simulink model "PESO_ex1"  (R2020b)
settings: Solver=VariableStepAuto  StartTime=0.0  StopTime=20  FixedStep=1e-6  RelTol=1e-4
settings Model: Creator=Amir  LastModifiedBy=Amir
settings DataIOCC: ReturnWorkspaceOutputs=off

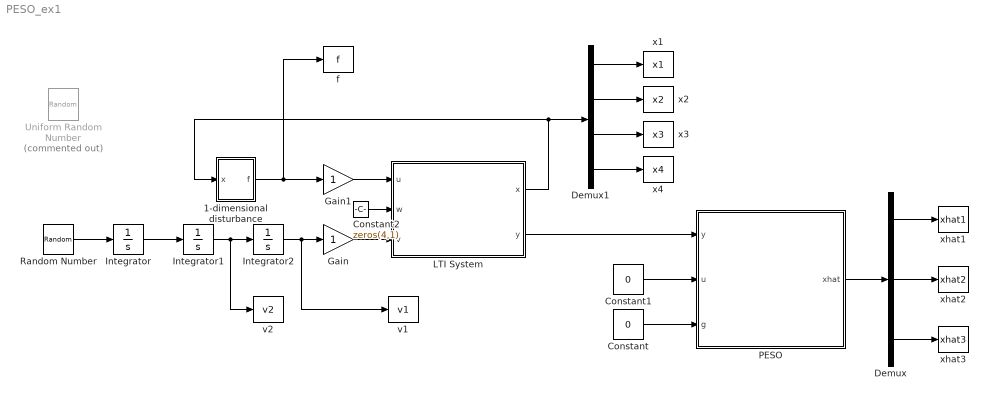
== system PESO_ex1 ==
  1-dimensional disturbance : Subsystem
  Constant : Constant  Value=0
  Constant1 : Constant  Value=0
  Constant2 : Constant  Value=zeros(4,1)
  Demux : Demux  Outputs=3
  Demux1 : Demux
  Gain : Gain
  Gain1 : Gain
  Integrator : Integrator
  Integrator1 : Integrator
  Integrator2 : Integrator
  LTI System : Subsystem  mask{n=4, m=1, k=1, A=[0 1 0 0;0 0 1 0;0 0 0 1;0 0 0 0], B=[0;0;0;1], C=[1 0 0 0], D=0, x0=[1;1;1;1]}
      mask prompts: n "Length of state vector (n):"; m "Length of input vector (m):"; k "Length of output vector (k):"; x0 "x(0):"
      mask DialogControl DescGroupVar Prompt: Main
      mask DialogControl DescTextVar Prompt: This block simulates a linear time-invariant (LTI) system. The system can be written as 'dx/dt=Ax+Bu+w' and 'y=Cx+Du+v'.
      mask DialogControl ParameterGroupVar Prompt: Dimensions
      mask DialogControl ParameterGroupVar_copy Prompt: Parameters
      mask DialogControl ParameterGroupVar_copy_copy Prompt: Initial Condition
  PESO : Subsystem  mask{n=2, tau=20, b=-[3;3;1], alpha=0.03, x0=10*[1;1], epsilon_t=1e-3}
      mask prompts: n "Dimension of the system (n):"; tau "Convergence time (tau):"; b "Vector of observer gains (b):"; alpha "Mapping gain (alpha):"; x0 "Initial Estimated state (x0):"; epsilon_t "Switching tolerance (epsilon_t):"
      mask DialogControl DescGroupVar Prompt: Main
      mask DialogControl DescTextVar Prompt: Prescribed-time observer for unknown systems.
  Random Number : RandomNumber  Variance=1e-6  SampleTime=1e-4
  Uniform Random Number : UniformRandomNumber  Commented=on  Minimum=-1e-3  Maximum=1e-3  Seed=-100  SampleTime=1e-4
  f : ToWorkspace  VariableName=f  SampleTime=-1
      settings: Save2DSignal=2-D array (concatenate along first dimension)
  v1 : ToWorkspace  VariableName=v1  SampleTime=-1
      settings: Save2DSignal=2-D array (concatenate along first dimension)
  v2 : ToWorkspace  VariableName=v2  SampleTime=-1
      settings: Save2DSignal=2-D array (concatenate along first dimension)
  x1 : ToWorkspace  VariableName=x1  SampleTime=-1
      settings: Save2DSignal=2-D array (concatenate along first dimension)
  x2 : ToWorkspace  VariableName=x2  SampleTime=-1
      settings: Save2DSignal=2-D array (concatenate along first dimension)
  x3 : ToWorkspace  VariableName=x3  SampleTime=-1
      settings: Save2DSignal=2-D array (concatenate along first dimension)
  x4 : ToWorkspace  VariableName=x4  SampleTime=-1
      settings: Save2DSignal=2-D array (concatenate along first dimension)
  xhat1 : ToWorkspace  VariableName=xhat1  SampleTime=-1
      settings: Save2DSignal=2-D array (concatenate along first dimension)
  xhat2 : ToWorkspace  VariableName=xhat2  SampleTime=-1
      settings: Save2DSignal=2-D array (concatenate along first dimension)
  xhat3 : ToWorkspace  VariableName=xhat3  SampleTime=-1
      settings: Save2DSignal=2-D array (concatenate along first dimension)
  wires:
  LTI System/2(y) -> PESO/1(y)
  PESO/1(xhat) -> Demux/1
  Demux/1 -> xhat1/1
  Demux/2 -> xhat2/1
  Demux/3 -> xhat3/1
  LTI System/1(x) -> Demux1/1, 1-dimensional disturbance/1(x)
  Demux1/1 -> x1/1
  Demux1/2 -> x2/1
  1-dimensional disturbance/1(f) -> Gain1/1, f/1
  Integrator/1 -> Integrator1/1
  Demux1/3 -> x3/1
  Demux1/4 -> x4/1
  Constant/1 -> PESO/3(g)
  Gain1/1 -> LTI System/1(u)
  Integrator2/1 -> v1/1, Gain/1
  Integrator1/1 -> v2/1, Integrator2/1
  Constant1/1 -> PESO/2(u)
  Constant2/1 -> LTI System/2(w)
  Gain/1 -> LTI System/3(v)
  Random Number/1 -> Integrator/1

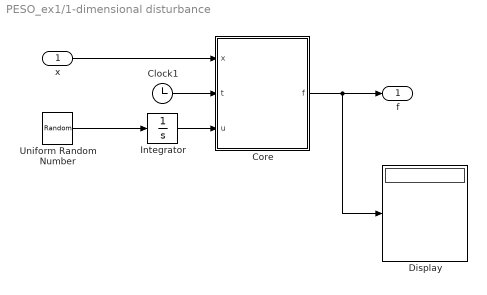
== system PESO_ex1/1-dimensional disturbance ==
  x : Inport
  Clock1 : Clock
  Core : MATLAB Function  TreatAsAtomicUnit=on
  Display : Display
  Integrator : Integrator
  Uniform Random Number : UniformRandomNumber  SampleTime=1e-4
  f : Outport
  wires:
  Core/1(f) -> f/1, Display/1
  Clock1/1 -> Core/2(t)
  x/1 -> Core/1(x)
  Uniform Random Number/1 -> Integrator/1
  Integrator/1 -> Core/3(u)

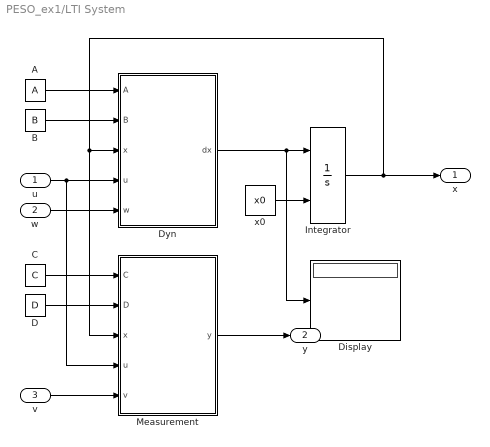
== system PESO_ex1/LTI System ==
  u : Inport
  w : Inport  Port=2
  v : Inport  Port=3
  A : Constant  Value=A
  B : Constant  Value=B
  C : Constant  Value=C
  D : Constant  Value=D
  Display : Display
  Dyn : MATLAB Function  TreatAsAtomicUnit=on
  Integrator : Integrator  InitialConditionSource=external
  Measurement : MATLAB Function  TreatAsAtomicUnit=on
  x0 : Constant  Value=x0
  x : Outport
  y : Outport  Port=2
  wires:
  v/1 -> Measurement/5(v)
  w/1 -> Dyn/5(w)
  u/1 -> Measurement/4(u), Dyn/4(u)
  Dyn/1(dx) -> Display/1, Integrator/1
  x0/1 -> Integrator/2
  B/1 -> Dyn/2(B)
  A/1 -> Dyn/1(A)
  C/1 -> Measurement/1(C)
  D/1 -> Measurement/2(D)
  Measurement/1(y) -> y/1
  Integrator/1 -> Measurement/3(x), Dyn/3(x), x/1

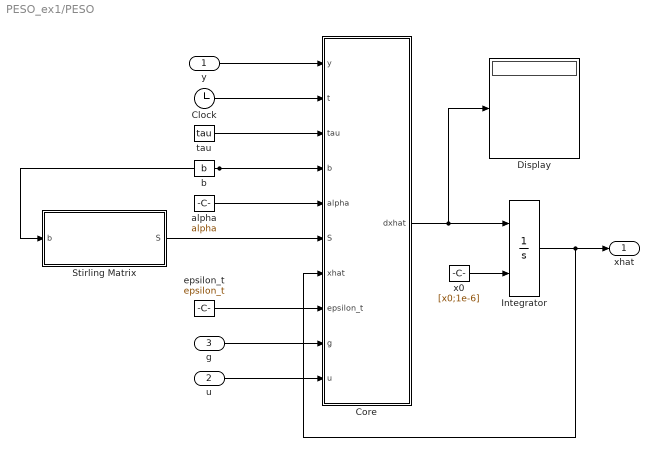
== system PESO_ex1/PESO ==
  y : Inport
  u : Inport  Port=2
  g : Inport  Port=3
  Clock : Clock
  Core : MATLAB Function  TreatAsAtomicUnit=on
  Display : Display
  Integrator : Integrator  InitialConditionSource=external
  Stirling Matrix : MATLAB Function  TreatAsAtomicUnit=on
  alpha : Constant  Value=alpha
  b : Constant  Value=b
  epsilon_t : Constant  Value=epsilon_t
  tau : Constant  Value=tau
  x0 : Constant  Value=[x0;1e-6]
  xhat : Outport
  wires:
  alpha/1 -> Core/5(alpha)
  b/1 -> Core/4(b), Stirling Matrix/1(b)
  y/1 -> Core/1(y)
  tau/1 -> Core/3(tau)
  Clock/1 -> Core/2(t)
  Stirling Matrix/1(S) -> Core/6(S)
  Core/1(dxhat) -> Display/1, Integrator/1
  x0/1 -> Integrator/2
  Integrator/1 -> xhat/1, Core/7(xhat)
  epsilon_t/1 -> Core/8(epsilon_t)
  u/1 -> Core/10(u)
  g/1 -> Core/9(g)

== matlab function PESO_ex1/LTI System/Measurement ==
  data: C input size=[k n]; D input size=[k m]; x input size=[n 1]; u input size=[m 1]; y output size=[k 1]; v input size=[k 1]
function y  = y_gen(C,D,x,u,v)

y = C*x+D*u+v;

== matlab function PESO_ex1/LTI System/Dyn ==
  data: A input size=[n n]; B input size=[n m]; x input size=[n 1]; u input size=[m 1]; dx output size=[n 1]; w input size=[n 1]
function dx  = dx_gen(A,B,x,u,w)

dx = A*x+B*u+w;

== matlab function PESO_ex1/1-dimensional disturbance/Core ==
  data: x input size=[4 1]; t input; u input; f output
function f = fcn(x,t,u)

f=(t^3+t^2+t+1)*(sin(x(1))+cos(x(1))+u);

== matlab function PESO_ex1/PESO/Core ==
  data: y input size=[1 1]; dxhat output size=[n+1 1]; t input size=[1 1]; tau input size=[1 1]; b input size=[n+1 1]; alpha input size=[1 1]; S input size=[n+2 n+2]; xhat input size=[n+1,1]; epsilon_t input; g input; u input
function dxhat = PTC_gen(y,t,tau,b,alpha,S,xhat,epsilon_t,g,u)

if t>tau-epsilon_t
    
    t=tau-epsilon_t;
    
end

n=length(b)-1;

dxhat=zeros(n+1,1);

p=zeros(n+1,1);

for i=1:n+1
    
    sum=0;
    
    for j=i:n+1
        
        sum=sum+S(j,i)*(b(n-j+2))*(-1)^(j-i)/(alpha^(n-j+2)*(tau-t)^(n-i+2));
        
    end
    
    p(n-i+2)=-S(n+2,i)*(-1)^(n-i+2)/(tau-t)^(n-i+2)+sum;
    
end

for i=1:n-1
    
    dxhat(i)=xhat(i+1)+p(i)*(xhat(1)-y);
    
end

dxhat(n)=xhat(n+1)+p(n)*(xhat(1)-y)+g*u;

dxhat(n+1)=p(n+1)*(xhat(1)-y);

== matlab function PESO_ex1/PESO/Stirling Matrix ==
  data: b input size=[n+1 1]; S output size=[n+2 n+2]
function S = Stirling_gen(b)

n=length(b)+1;

S=zeros(n,n);

for i=1:n
    
    for j=1:n
        
        if i>=j
            
            m=0;

            for l=0:j-1
    
                sum=1/factorial(j-1)*(-1)^l*(factorial(j-1)/(factorial(l)*factorial(j-1-l)))*(j-1-l)^(i-1);
                
                m=m+sum;
                
            end
            
            S(i,j)=m;
            
        end
        
    end
    
end
